simulink model "test_on_cm_lon_lat"  (R2019b)
settings: Solver=FixedStepAuto  StartTime=0.0  StopTime=10.0  FixedStep=0.01  RelTol=1e-3
settings Model: Creator=lenovo  LastModifiedBy=lenovo

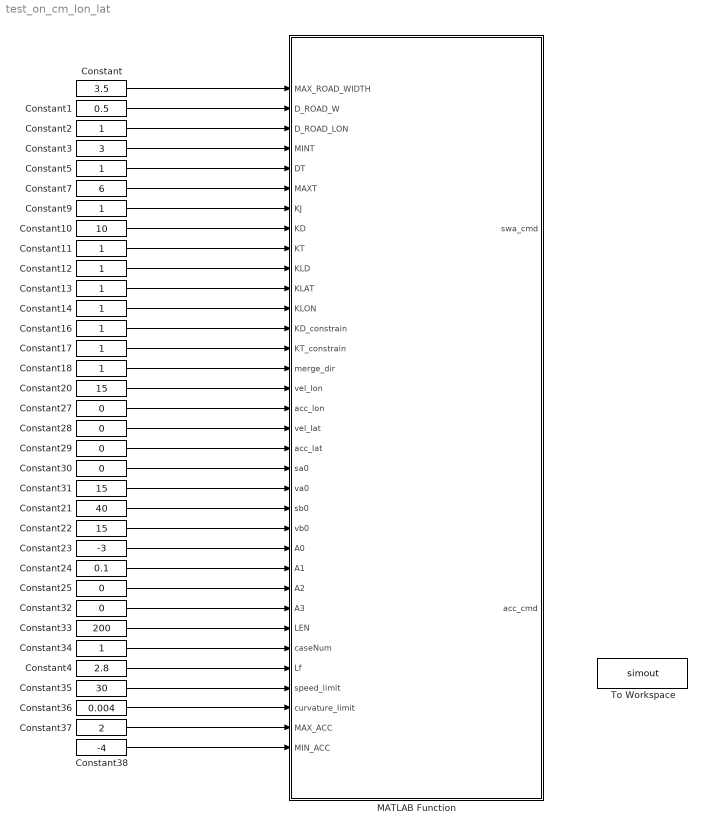
== system test_on_cm_lon_lat ==
  Constant : Constant  Value=3.5
  Constant1 : Constant  Value=0.5
  Constant10 : Constant  Value=10
  Constant{2,5,9,11..14,16..18,34} (11 alike) : Constant
  Constant20 : Constant  Value=15
  Constant21 : Constant  Value=40
  Constant22 : Constant  Value=15
  Constant23 : Constant  Value=-3
  Constant24 : Constant  Value=0.1
  Constant{25,27..30,32} (6 alike) : Constant  Value=0
  Constant3 : Constant  Value=3
  Constant31 : Constant  Value=15
  Constant33 : Constant  Value=200
  Constant35 : Constant  Value=30
  Constant36 : Constant  Value=0.004
  Constant37 : Constant  Value=2
  Constant38 : Constant  Value=-4
  Constant4 : Constant  Value=2.8
  Constant7 : Constant  Value=6
  MATLAB Function : MATLAB Function  TreatAsAtomicUnit=on
  To Workspace : ToWorkspace  VariableName=simout  SaveFormat=Structure  SampleTime=-1
  wires:
  Constant/1 -> MATLAB Function/1(MAX_ROAD_WIDTH)
  Constant1/1 -> MATLAB Function/2(D_ROAD_W)
  Constant2/1 -> MATLAB Function/3(D_ROAD_LON)
  Constant3/1 -> MATLAB Function/4(MINT)
  Constant5/1 -> MATLAB Function/5(DT)
  Constant7/1 -> MATLAB Function/6(MAXT)
  Constant9/1 -> MATLAB Function/7(KJ)
  Constant10/1 -> MATLAB Function/8(KD)
  Constant11/1 -> MATLAB Function/9(KT)
  Constant12/1 -> MATLAB Function/10(KLD)
  Constant13/1 -> MATLAB Function/11(KLAT)
  Constant14/1 -> MATLAB Function/12(KLON)
  Constant16/1 -> MATLAB Function/13(KD_constrain)
  Constant17/1 -> MATLAB Function/14(KT_constrain)
  Constant18/1 -> MATLAB Function/15(merge_dir)
  Constant20/1 -> MATLAB Function/16(vel_lon)
  Constant27/1 -> MATLAB Function/17(acc_lon)
  Constant28/1 -> MATLAB Function/18(vel_lat)
  Constant29/1 -> MATLAB Function/19(acc_lat)
  Constant30/1 -> MATLAB Function/20(sa0)
  Constant31/1 -> MATLAB Function/21(va0)
  Constant21/1 -> MATLAB Function/22(sb0)
  Constant22/1 -> MATLAB Function/23(vb0)
  Constant23/1 -> MATLAB Function/24(A0)
  Constant24/1 -> MATLAB Function/25(A1)
  Constant25/1 -> MATLAB Function/26(A2)
  Constant32/1 -> MATLAB Function/27(A3)
  Constant33/1 -> MATLAB Function/28(LEN)
  Constant34/1 -> MATLAB Function/29(caseNum)
  Constant35/1 -> MATLAB Function/31(speed_limit)
  Constant36/1 -> MATLAB Function/32(curvature_limit)
  Constant37/1 -> MATLAB Function/33(MAX_ACC)
  Constant38/1 -> MATLAB Function/34(MIN_ACC)
  ? -> To Workspace/1
  Constant4/1 -> MATLAB Function/30(Lf)

== matlab function test_on_cm_lon_lat/MATLAB Function ==
  data: swa_cmd output; acc_cmd output; MAX_ROAD_WIDTH input; D_ROAD_W input; D_ROAD_LON input; MINT input; DT input; MAXT input; KJ input; KD input; KT input; KLD input; KLAT input; KLON input; KD_constrain input; KT_constrain input; merge_dir input; vel_lon input; acc_lon input; vel_lat input; acc_lat input; sa0 input; va0 input; sb0 input; vb0 input; A0 input; A1 input; A2 input; A3 input; LEN input; caseNum input; Lf input; speed_limit input; curvature_limit input; MAX_ACC input; MIN_ACC input
























function [swa_cmd,acc_cmd] = dynamic_planning(MAX_ROAD_WIDTH,D_ROAD_W,D_ROAD_LON,...
    MINT, DT, MAXT, KJ, KD, KT, KLD, KLAT, KLON, KD_constrain, KT_constrain, ...
    merge_dir, vel_lon, acc_lon, vel_lat, acc_lat,...
    sa0, va0, sb0, vb0,...
    A0, A1, A2, A3,...
    LEN, caseNum, Lf,...
    speed_limit, curvature_limit, MAX_ACC, MIN_ACC)
    %% this function discrriminate two different sampling methods.
    % if caseNum ==4, it means this is simple lane changing, we change lane
    % without considering of velocity planning
    % if caseNum != 4, it means this is merging lane changing, we apply
    % x(t)-y(t) method to plan spatially and temporally. 
    
 
    [reference] = reference_line_generator(A0,A1,A2,A3);
   
        % do merging method lane changing
        
        [cost_graph] = calc_frenet_paths_constraint(MAX_ROAD_WIDTH, D_ROAD_W, D_ROAD_LON, MINT, DT, MAXT,...
            KJ, KLD, KLAT, KLON, KD_constrain, KT_constrain,...
            merge_dir, vel_lon, acc_lon, vel_lat, acc_lat,...
            sa0, va0, sb0, vb0,...
            A0, A1, A2, A3,...
            LEN, caseNum);
        
        cost_graph_optimal = check_status(cost_graph,speed_limit,MAX_ACC,MIN_ACC,curvature_limit);
        [y_of_x,p_of_v,p_of_a] = conbination(cost_graph_optimal);
        
        [ref_poly] = ref_poly_generation(reference, y_of_x);
        
%         figure
%         plot(ref_poly(:,1),ref_poly(:,2));
        
        
        trajs_new_origin = reference_generation(reference, ref_poly);% 
        
        figure
        plot(trajs_new_origin(:,1),trajs_new_origin(:,2));
        hold on
        plot(reference(:,1),reference(:,2));
        
        [len_valid_data] = find_valid_ref_max_len(y_of_x);
        [v_profile] = velocity_intepolation(p_of_v,reference,len_valid_data);
        [a_profile] = acc_intepolation(p_of_a,reference,len_valid_data);
        delta_heading_rad = calculat_delta_heading(reference, trajs_new_origin);
        delta_heading_deg = rad_to_deg(delta_heading_rad); % If you need 
        kappa = calculate_kappa_oneshot(trajs_new_origin);
        
       
        
        [ref_point,swa_cmd] = calculate_swa_cmd(trajs_new_origin,vel_lon,Lf);
        acc_cmd = a_profile(20,2);
%         output = transition_to_BUS(output);

end 


function [ref_point,swa_cmd] = calculate_swa_cmd(trajs_new_origin,vel_lon,Lf)
    if vel_lon < 5
        constDist = 18;
    else
        constDist = 9;
    end
    distPre = min(0.5 * vel_lon+constDist, 18);
    
    S = 0;
    ind = 1;
    while ind < length(trajs_new_origin) && S < distPre
        S = S + norm(trajs_new_origin(ind+1,:)-trajs_new_origin(ind,:));
        ind = ind + 1;
    end
    ref_point = trajs_new_origin(ind-1 ,:);
    
    preview_dist  = norm(ref_point);
    preview_angle = atan(ref_point(2)/ref_point(1));
    swa_cmd = atan(2 * Lf * sin(preview_angle) / preview_dist) * 180 / pi; % cmd in deg unit.
%% 
end
%
function [v_profile] = velocity_intepolation(p_of_v,reference,len_valid_data)
    
S = 0;
    v_profile = [];
    index =1;
    X = p_of_v(1:len_valid_data,1);
    V = p_of_v(1:len_valid_data,3);
    XMAX = min(reference(end,1),X(end));
    
    while S <= XMAX && (index+1) <= length(reference)
        
        v = [S,interp1(X,V,S,'spline')];
        
        v_profile =[v_profile; v];
        S = S + sqrt((reference(index+1,1)-reference(index,1))^2 + ...
            (reference(index+1,2)-reference(index,2))^2);
        index = index + 1;
    end


end
%
function [a_profile] = acc_intepolation(p_of_a,reference,len_valid_data)
    
    S = 0;
    a_profile = [];
    index =1;
    X = p_of_a(1:len_valid_data,1);
    A = p_of_a(1:len_valid_data,3);
    XMAX = min(reference(end,1),X(end));
    
    while S <= XMAX && (index+1) <= length(reference)
        
        a = [S,interp1(X,A,S,'spline')];
        
        a_profile =[a_profile; a];
        S = S + sqrt((reference(index+1,1)-reference(index,1))^2 + ...
            (reference(index+1,2)-reference(index,2))^2);
        index = index + 1;
    end
end
%
function [ref_poly] = ref_poly_generation(reference, y_of_x)
%% this function generate polynomial curve informaion, in this function, we find 
%% according to the reference line, the lateral offset 
    S = 0;
    ref_poly = zeros(400,2);
    index = 1;
    [len_valid] = find_valid_ref_max_len(y_of_x);
    X = y_of_x(1:len_valid,1);
    Y = y_of_x(1:len_valid,2);
    XMAX = min(reference(end,1),X(end));
    
    while S <= XMAX && (index+1) <= length(reference)
        
        p = [S,interp1(X,Y,S,'spline')];
        
        ref_poly(index,:) = p;
        S = S + sqrt((reference(index+1,1)-reference(index,1))^2 + ...
            (reference(index+1,2)-reference(index,2))^2);
        index = index + 1;
    end
    
     [len_valid_poly] = find_valid_ref_max_len(ref_poly);
     ref_poly = ref_poly(1:len_valid_poly-1,:);
end
%
function [y_of_x,p_of_v,p_of_a] = conbination(frenet_data)
    Te = frenet_data(2);  
    a = zeros(1,6);
    b = zeros(1,6);
    delta_t = 0.025;
    
    SIZE = Te / delta_t;
   
    for i = 5:10
        a(i-4) = frenet_data(i);
        b(i-4) = frenet_data(i+6);
    end
    
    yt = zeros(1,400);
    vyt= zeros(1,400);
    ayt= zeros(1,400);
    xt = zeros(1,400);
    vxt= zeros(1,400);
    axt= zeros(1,400);
    
    a0 = a(1); a1 = a(2); a2 = a(3); a3 = a(4);
    a4 = a(5); a5 = a(6); b0 = b(1); b1 = b(2);
    b2 = b(3); b3 = b(4); b4 = b(5); b5 = b(6);  
   
        
    for ind = 1: SIZE+1
        t = (ind-1) * delta_t;
        yt(ind) = calc_point(a0,a1,a2,a3,a4,a5,t);
        vyt(ind) = calc_first_derivative(a1,a2,a3,a4,a5,t);
        ayt(ind) = calc_second_derivative(a2,a3,a4,a5,t);
        xt(ind) = calc_point(b0,b1,b2,b3,b4,b5,t);
        vxt(ind) = calc_first_derivative(b1,b2,b3,b4,b5,t);
        axt(ind) = calc_second_derivative(b2,b3,b4,b5,t);
        
    end
    
    velocity = sqrt(vxt.^2 + vyt.^2);
    acceleration = axt; %sign(axt).* sqrt(axt.^2 + ayt.^2);
    y_of_x = [xt',yt'];
    p_of_v = [xt',yt',velocity'];
    p_of_a = [xt',yt',acceleration'];
    

end


function [len_valid] = find_valid_ref_max_len(reference)
    pos = find(reference(:,1)==0 & reference(:,2) == 0);
    if length(pos) == 1
        len_valid = length(reference)-1;
        
    else
        if pos(1) == 1
            len_valid = pos(2)-1;
        else
            len_valid = pos(1)-1;
        end
    end
    
end
%%
function cost_graph_optimal = check_status(cost_graph,speed_limit,MAX_ACC,MIN_ACC,curvature_limit)
 
    i = 1;
    COND = 1;
    a = zeros(1,6);
    b = zeros(1,6);
    cost_graph_optimal = zeros(1,16);
    
    while COND == 1
        frenet_data = cost_graph(i,:);
        Te = frenet_data(2);        
        for j = 5:10
            a(j-4) = frenet_data(j);
            b(j-4) = frenet_data(j+6);
        end
    
        xt = [];
        yt = [];
        vxt = [];
        vyt = [];
        axt = [];
        ayt = [];

        for t = 0:0.4:Te
            a0 = a(1); a1 = a(2); a2 = a(3); a3 = a(4);
            a4 = a(5); a5 = a(6); b0 = b(1); b1 = b(2);
            b2 = b(3); b3 = b(4); b4 = b(5); b5 = b(6);
            [yt] = [yt,calc_point(a0,a1,a2,a3,a4,a5,t)];
            [vyt] = [vyt, calc_first_derivative(a1,a2,a3,a4,a5,t)];
            [ayt] = [ayt, calc_second_derivative(a2,a3,a4,a5,t)];
            [xt] = [xt, calc_point(b0,b1,b2,b3,b4,b5,t)];
            [vxt] =[ vxt, calc_first_derivative(b1,b2,b3,b4,b5,t)];
            [axt] = [axt, calc_second_derivative(b2,b3,b4,b5,t)];
        end
        
        trajs = [xt',yt'];
        velocity = sqrt(vxt.^2 + vyt.^2);
        acceleration = sign(axt) .* sqrt(axt.^2 + ayt.^2);
        kappa = calculate_kappa_oneshot(trajs);
        
        if ((max(abs(velocity))<= speed_limit) && (max(acceleration)<=MAX_ACC)...
                && (min(acceleration) >= MIN_ACC) && (max(abs(kappa)) < curvature_limit))
            cost_graph_optimal = cost_graph(i,:);
            COND = 2;
        end
        
        i = i+1;
        
        if  i > size(cost_graph,1)
            COND = 2;
            cost_graph_optimal = cost_graph(1,:);
        end
    end
        
        
end
%%
function [cost_graph] = calc_frenet_paths_constraint(MAX_ROAD_WIDTH, D_ROAD_W, D_ROAD_LON, MINT, DT, MAXT,...
    KJ, KLD, KLAT, KLON, KD_constrain, KT_constrain,...
    merge_dir, vel_lon, acc_lon, vel_lat, acc_lat,...
    sa0, va0, sb0, vb0,...
    A0, A1, A2, A3,...
    LEN, caseNum)

% @breif this is the function to sample all possible candidate in cases of
    % constrained merging scenarios. it uses x(t)-y(t) method, which means it
    % outputs spatial and temporal profiles.

% input: 
    % directly call all global data
    
% output:
    % cost graph maintains all sampled candidate information, which is as
    % follow: The first col is the total cost. The second col is Ti, which
    % is time T. The third col is di, which is terminal lateral offset. The
    % fourth col is si, which is terminal longitudinal distance.  
        
    frenet_paths =[]; % initiate it with empty
    cost_graph = []; % initiate it with empty
    
    if merge_dir == 1 % merging to left lane
        lower_bound = -MAX_ROAD_WIDTH / 2;
        upper_bound = 0;
    else % merging to right lane
        lower_bound = 0;
        upper_bound = MAX_ROAD_WIDTH / 2;
    end
    
    for Ti = MINT : DT : MAXT
        for di = lower_bound : D_ROAD_W : upper_bound
            xs = A0;
            vxs = vel_lat;
            axs = acc_lat;
            %Ti is sampling on T
            xe = di; % sampling on lateral offset
            vxe = 0;
            axe = 0;
            [a0, a1, a2, a3, a4,a5] = quintic_polynomial(xs, ...
                vxs, axs, xe, vxe, axe,Ti);
            [jerk_bar_lat] = cal_j_bar(a3,a4,a5,Ti);
            [d_bar_lat] = calc_d_bar(a0,a1,a2,a3,a4,a5,Ti);
            cost_total_lat = KJ * jerk_bar_lat + KD_constrain * d_bar_lat + KT_constrain * Ti;
            
            
            xs = 0;
            vxs = vel_lon;
            axs = acc_lon;

            [xe,sa,sb] = cal_xe(caseNum, sa0,sb0,va0,vb0,Ti); % go to function definition for details
            
            delta_s = 1/4 * (sb - sa); % how to determine ??? we still have not make sure 
            
            vxe = 1/2 * (va0 + vb0);
            axe = 0;
            
            for si = xe - delta_s : D_ROAD_LON : xe + delta_s
           
                [b0, b1, b2, b3, b4, b5] = quintic_polynomial(xs, ...
                    vxs, axs, xe, vxe, axe,Ti);
                [jerk_bar_lon] = cal_j_bar(b3,b4,b5,Ti);
                delta_d = abs(si - xe);

                cost_total_lon = KJ * jerk_bar_lon + KLD * delta_d + KT_constrain * Ti;
               
                cost_total = KLAT * cost_total_lat + KLON * cost_total_lon;
                cost_graph = [cost_graph;[cost_total, Ti, di, si,...
                    a0, a1, a2, a3, a4, a5, b0, b1, b2, b3, b4, b5]];
            end
        end
    end
    cost_graph = sortrows(cost_graph);
end

%%
function [a0, a1, a2, a3, a4,a5] = quintic_polynomial(xs, ...
    vxs, axs, xe, vxe, axe,T)
% A = [0,0,0,0,0,1; T^5,T^4,T^3,T^2,T,1;...
%     0,0,0,0,1,0 ; 5*T^4  4*T^3 3*T^2 2*T 1 0 ; ...
%     0 0 0 2 0 0; 20*T^3 12*T^2 6*T 2 0 0];
% b = [xs, xe, vxs, vxe, axs, 0]';
% x = A\b;
% a5 = x(1);
% a4 = x(2);
% a3 = x(3);
% a2 = x(4);
% a1 = x(5);
% a0 = x(6);
A = [T^3 T^4 T^5; 3*T^2 4*T^3 5*T^4; 6*T 12*T^2 20*T^3];
b = [(xe - xs  - vxs*T - 0.5*axs*T^2); (vxe- vxs - axs*T ); (axe - axs)];
x = A\b;
a0 = xs;
a1 = vxs;
a2 = axs/2;

a3 = x(1);
a4 = x(2);
a5 = x(3);
end

function [xt] = calc_point(a0,a1,a2,a3,a4,a5,t)
xt = a0 + a1 * t + a2 * t ^2 + a3 * t^3 + a4 * t^4 + a5 * t^5;
end

function [d_bar] = calc_d_bar(a0,a1,a2,a3,a4,a5,T)
    xt = [];
    for t =0 : 0.4 : T
        xt = [xt, calc_point(a0,a1,a2,a3,a4,a5,t)];
    end
    d_bar = mean(abs(xt));
end

function [jerk_bar] = cal_j_bar(a3,a4,a5,T)
    jt = [];
    for t =0 : 0.4 : T
        jt = [jt, calc_third_derivative(a3,a4, a5,t)];
    end
    jerk_bar = mean(abs(jt));
end

function [xe,sa,sb] = cal_xe(caseNum, sa0,sb0,va0,vb0,Ti)
    CONST =60; % It remains uncertain how how to choose a properiate distance CONST.    
    switch caseNum
        case 1 % in this case, we have vehicle a and vehilce b;
            sa = sa0 + va0 * Ti; % a_vehicle: the nearest adjacent vehicle which is declared as rear vehicle;
            sb = sb0 + vb0 * Ti; % b_vehilce: the nearest adjacent vehicle that is in front of the a_vehicle(front vehicle);
            xe = sa + (sb - sa) * 2/3;% 1/2 * (sb + sa);
        case 2 % in this case, we have only vehicle a;
           sa = sa0 + va0 * Ti;
           sb = sa + CONST; % the distance between two vehicles is CONST
           xe = sa + (sb - sa) * 2/3;% 1/2 * (sb + sa);
        otherwise % in this case, we only have vehicle b;
           sb = sb0 + vb0 * Ti;
           sa =  sb - CONST; % the distance between two vehicles is CONST
           xe = sa + (sb - sa) * 2/3;% 1/2 * (sb + sa);
    end              
end
%  
function [reference] = reference_line_generator(a0,a1,a2,a3)
%% in this function, we use the left and right lane polynomials to generate
% a reference center line
% input: left lane polynomials, right lane polynomials, LEN(length of reference)
% output: reference center line polynomials
reference = zeros(400, 2);


for i =1 : 400
    x = 0.5 * (i-1);
    y = 0.5 * (a0 + a1 * x + a2 * x^2 + a3 * x^3);
    reference(i,:) = [x,y];
end

end
%%
function y = f_a(a0, a1, a2, a3, x)
%% calculate polynomial y values
    y = a0 + a1 * x + a2 * x^2 + a3 * x^3;
end

function y = f_b(b0, b1, b2, b3, x)
%% calculate polynomial y values
    y = b0 + b1 * x + b2 * x^2 + b3 * x^3;
end

function y = deg_to_rad(x)
%% deg to rad unit switch
    y = x * pi / 180;
end

function y = rad_to_deg(x)
%% rad to degree unit switch
    y = x * 180 / pi;
end

function [trajs_new] = reference_generation(trajs_local, p_store)
%% this function provides method of generating changing lane discrete positions.    
% inputs: here the trajs_local is a vector<vector<double>>,with its dimension
%n by 2, the p_store store the information Bezier curve generaion
%function creates, which are longitudinal 's' and 'lateral offset', which
%is also in dimension of n by 2. 
%output: with the two inputs info, we are able to generate under vehicle
%coordinate the changing lane positions by doing position shift, based on
%the original trajs_local, in frenet direction with offset info provided by
%p_store.


    trajs_new = zeros(400,2);
    for i = 1: length(p_store)
%         if (i + current_index) > length(waypoint)
%             break;
        d = p_store(i,2);
        if trajs_local(i,1) == 0
            theta = 0;
        elseif (i == 1)
            theta = atan(trajs_local(i,2) / trajs_local(i,1)+0.001);
        else
            theta = atan((trajs_local(i,2) - trajs_local(i-1,2)) / (trajs_local(i,1) - trajs_local(i-1,1)));
        end
        
        if (theta>-pi/2 && theta <=0)
            x = trajs_local(i,1) + d * sin(theta);
            y = trajs_local(i,2) + d * cos(theta);
            trajs_new(i,:) = [x,y];
        elseif (theta>0 && theta < pi/2)
            x = trajs_local(i,1) - d * sin(theta);
            y = trajs_local(i,2) + d * cos(theta);
            trajs_new(i,:) = [x,y];    
        else
           fprintf("it seems that the reference line is unacceptable!");
        end
    end
    
     [len_valid_traj] = find_valid_ref_max_len(trajs_new);
     trajs_new = trajs_new(1:len_valid_traj-1,:);
end

%%
function [k] = calculate_kappa(p,pd,pdd) 
     for i  = 1:length(p)
         k(i) = (pdd(i))/((1+pd(i)^2)^(1.5));
     end
end

%%
function [pd] = calculate_pd(p)
    % calculate the first derivatives
    pd = zeros(length(p),1);
    for i = 1:length(p)-1
     pd(i) = (p(i+1,2)-p(i,2))/(p(i+1,1)-p(i,1));
    end
end

%%
function [pdd] = calculate_pdd(p)
    % calculate the second derivatives
     pdd = zeros(length(p),1);
     for i =2: length(p)-1
         pdd(i) = (p(i+1,2)-2*p(i,2) + p(i-1,2))/(0.5*(-p(i-1,1)+p(i+1,1)))^2;
    %    pdd(i) = (p(i+1,2)-2*p(i,2) + p(i-1,2))/(-p(i,1)+p(i+1,1))^2;
     end
end

%%
function [kappa_d] = calculate_kappa_d(p,k)
    kappa_d = zeros(length(p),1);
    kappa_d(1) = 0;
    for i = 2: length(p)
        kappa_d(i) = (k(i)-k(i-1))/norm(p(i,:)- p(i-1,:));
    end
end

%%
function [xt] =calc_first_derivative(a1,a2,a3,a4,a5,t)
xt = a1 + 2 * a2 * t + 3 * a3 * t^2 + 4 * a4 * t^3  +  5 * a5 * t^4;
end

%%
function [xt]  = calc_second_derivative(a2,a3,a4,a5,t)
xt = 2* a2 + 6* a3 * t + 12 * a4 * t^2 + 20* a5 *t^3;
end

%%
function [xt] = calc_third_derivative(a3,a4,a5,t)
xt =6 * a3 + 24 * a4 * t + a5 * t^2;
end

function [delta_heading] = calculat_delta_heading(center_line, traj_new)
    LEN = min(length(center_line), length(traj_new));
    delta_heading = [0];
    for i = 1: LEN-1
        x1 = center_line(i+1,1) - center_line(i,1);
        y1 = center_line(i+1,2) - center_line(i,2);
        x2 = traj_new(i+1,1) - traj_new(i,1);
        y2 = traj_new(i+1,2) - traj_new(i,2);
        delta_theta =  (x1 * x2 + y1 * y2) / (sqrt(x1^2 + y1^2) * sqrt(x2^2 + y2^2));
        delta_heading =  [delta_heading; acos(delta_theta)];
    end
end
%%

function [kappa] = calculate_kappa_oneshot(trajs_new)

% this function provide the method of generating a sequence of curvature(kappa) 
% input: a sequence of discrete points with position x and y.
% output: a sequence of kappa on each point.
% notice: vehicle turning right has negative curvature, and vice versa.

if (isempty(trajs_new)) || (length(trajs_new) == 0)
    fprintf('changing lane trajs is not well generated! \r');
    kappa = zeros(length(trajs_new),1);
    return;
end

    pd = zeros(length(trajs_new),1);
    pdd = zeros(length(trajs_new),1);
    kappa = zeros(length(trajs_new),1);
    
    % calculate the first derivatives
    
    for i = 1:length(trajs_new)-1
        
        if (trajs_new(i+1,1)-trajs_new(i,1)) == 0
            denominator_pd = 0.001;
        else
            denominator_pd = trajs_new(i+1,1)-trajs_new(i,1);
        end
        
        pd(i) = (trajs_new(i+1,2)-trajs_new(i,2))/denominator_pd;   
    end
    pd(length(trajs_new)) = pd(length(trajs_new)-1);
    % calculate the second derivatives
    pdd(1) = 0;
    for i =2: length(trajs_new)-1
        
        if (0.5*(-trajs_new(i-1,1)+trajs_new(i+1,1)))^2 == 0
            denominator_pdd = 0.001;
        else
            denominator_pdd = 0.5*(-trajs_new(i-1,1)+trajs_new(i+1,1))^2;
        end
        
        pdd(i) = (trajs_new(i+1,2)-2*trajs_new(i,2) +...
            trajs_new(i-1,2))/denominator_pdd;
    end
    pdd(length(trajs_new)) = pdd(length(trajs_new)-1);
    
    for i  = 1:length(trajs_new)
        kappa(i) = (pdd(i))/((1+pd(i)^2)^(1.5));
    end
end
